simulink model "qmult_test1"  (Simulink 7.0)
settings: Solver=FixedStepDiscrete  StartTime=0.0  StopTime=stop_time  FixedStep=1.0  RelTol=1e-3
libraries: simulink x4
Description:
  | Timing Test: Quaternion Multiplication, method 1
  | 
  | Copyright (c) 2001-2009, Jay A. St. Pierre.  All rights reserved.
settings Model: Creator=stpierre  LastModifiedBy=stpierre  ExtModeTrigMode=oneshot  ExtModeArmWhenConnect=off  ExtModeAutoUpdateStatusClock=off
settings DataIOCC: MaxDataPoints=1  SaveOutput=off  SaveTime=off
settings OptimizationCC: BlockReduction=off  BooleanDataType=off
settings DebuggingCC: SaveWithParameterizedLinksMsg=none  SignalResolutionControl=TryResolveAllWithWarning  SolverPrmCheckMsg=none  MultiTaskDSMMsg=warning  MultiTaskCondExecSysMsg=none  StrictBusMsg=None
settings HardwareCC: TargetUnknown=on
settings RTWCC: IncludeERTFirstTime=on

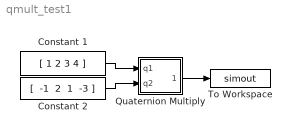
== system qmult_test1 ==
  Constant 1 : Constant  Value=[ 1 2 3 4 ]
  Constant 2 : Constant  Value="[  -1  2  1  -3 ]"
  Quaternion Multiply : Subsystem
      mask Type: Quaternion Multiply
      mask Description: q3 = (q1)(q2)
  To Workspace : ToWorkspace  VariableName=simout  SampleTime=-1  SaveFormat=Array
      settings: MaxDataPoints=1
  wires:
  Constant 1/1 -> Quaternion Multiply/1(q1)
  Quaternion Multiply/1(q1q2) -> To Workspace/1
  Constant 2/1 -> Quaternion Multiply/2(q2)

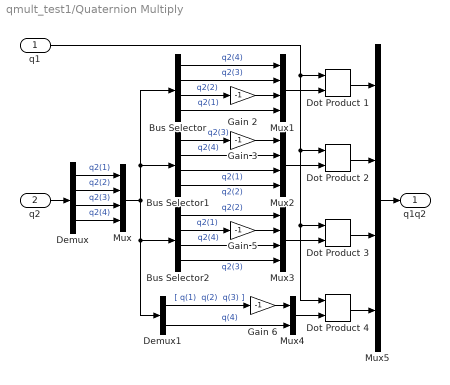
== system qmult_test1/Quaternion Multiply ==
  q1 : Inport  PortDimensions=4
  q2 : Inport  Port=2  PortDimensions=4
  Bus Selector : BusSelector  OutputSignals=q2(4),q2(3),q2(2),q2(1)
  Bus Selector1 : BusSelector  OutputSignals=q2(3),q2(4),q2(1),q2(2)
  Bus Selector2 : BusSelector  OutputSignals=q2(2),q2(1),q2(4),q2(3)
  Demux : Demux
  Demux1 : Demux  Outputs=[3 1]
  Dot Product {1..4} (4 alike) : simulink/Math Operations/Dot Product  InputSameDT=on  OutDataType=sfix(16)  OutScaling=2^-10  DoSatur=off
  Gain {2..3,5..6} (4 alike) : Gain  Gain=-1  SaturateOnIntegerOverflow=on
  Mux{,1..3,5} (5 alike) : Mux
  Mux4 : Mux  Inputs=2
  q1q2 : Outport  InitialOutput=0
  wires:
  Demux/4 -> Mux/4  "q2(4)"
  Demux/3 -> Mux/3  "q2(3)"
  Demux/2 -> Mux/2  "q2(2)"
  Demux/1 -> Mux/1  "q2(1)"
  q2/1 -> Demux/1
  Mux/1 -> Bus Selector1/1, Bus Selector/1, Bus Selector2/1, Demux1/1
  Dot Product 2/1 -> Mux5/2
  Mux5/1 -> q1q2/1
  Dot Product 4/1 -> Mux5/4
  Dot Product 3/1 -> Mux5/3
  Dot Product 1/1 -> Mux5/1
  q1/1 -> Dot Product 4/1, Dot Product 3/1, Dot Product 2/1, Dot Product 1/1
  Mux3/1 -> Dot Product 3/2
  Mux2/1 -> Dot Product 2/2
  Mux1/1 -> Dot Product 1/2
  Bus Selector2/3 -> Mux3/3  "q2(4)"
  Bus Selector1/2 -> Mux2/2  "q2(4)"
  Bus Selector/1 -> Mux1/1  "q2(4)"
  Bus Selector/2 -> Mux1/2  "q2(3)"
  Bus Selector/3 -> Gain 2/1  "q2(2)"
  Gain 2/1 -> Mux1/3
  Bus Selector/4 -> Mux1/4  "q2(1)"
  Bus Selector1/1 -> Gain 3/1  "q2(3)"
  Gain 3/1 -> Mux2/1
  Bus Selector1/3 -> Mux2/3  "q2(1)"
  Bus Selector1/4 -> Mux2/4  "q2(2)"
  Bus Selector2/2 -> Gain 5/1  "q2(1)"
  Gain 5/1 -> Mux3/2
  Bus Selector2/1 -> Mux3/1  "q2(2)"
  Bus Selector2/4 -> Mux3/4  "q2(3)"
  Mux4/1 -> Dot Product 4/2
  Demux1/1 -> Gain 6/1  "[ q(1)  q(2)  q(3) ]"
  Gain 6/1 -> Mux4/1
  Demux1/2 -> Mux4/2  "q(4)"
